simulink subsystem "forces"  (R2020a)
settings: Solver=VariableStepAuto  StartTime=0.0  StopTime=10.0  RelTol=1e-3
settings Model: Creator=Philip  LastModifiedBy=Philip

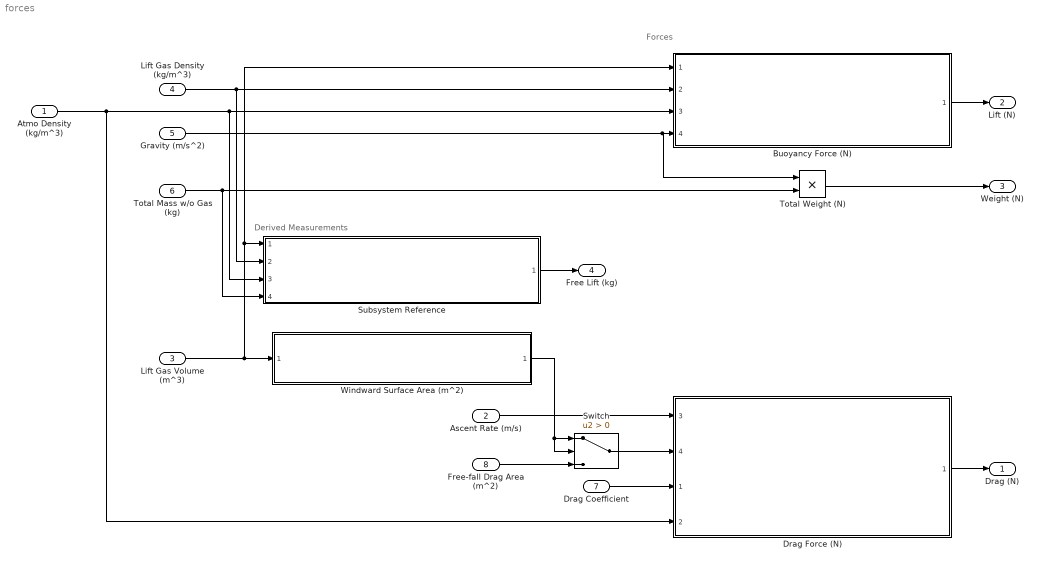
== system forces ==
  note: Forces
  note: Derived Measurements
  Atmo Density (kg/m^3) : Inport
  Ascent Rate (m/s) : Inport  Port=2
  Lift Gas Volume (m^3) : Inport  Port=3
  Lift Gas Density (kg/m^3) : Inport  Port=4
  Gravity (m/s^2) : Inport  Port=5
  Total Mass w/o Gas (kg) : Inport  Port=6
  Drag Coefficient : Inport  Port=7
  Free-fall Drag Area (m^2) : Inport  Port=8
  Buoyancy Force (N) : Subsystem  ReferencedSubsystem=buoyancy_force
  Drag Force (N) : Subsystem  ReferencedSubsystem=balloon_drag
      settings: PortSchema="{\"entries\":[{\"content\":{\"sides\":[{\"content\":{\"connectorIds\":[\"In3\",\"In4\",\"In1\",\"In2\"]},\"type\":\"ConnectorPlacement.EquallySpacedRectSide\",\"uuid\":\"149b4cde-76c5-4ca0-ad35-e24c4ea63904\"},{\"content\":{\"connectorIds\":[\"Out1\"],\"side\":\"RIGHT\"},\"type\":\"ConnectorPlacement.EquallySpacedRectSide\",\"uuid\":\"b3094bd8-666c-4796-b5f6-a24ca14a0216\"},{\"content\":{\"connectorIds\":[],\"side\":\"TOP\"},\"type\":\"ConnectorPlacement.EquallySpacedRectSide\",\"uuid\":\"8ef90c1d-a1d6-4cd7-a7b0-0fd7a3183b9f\"}]},\"type\":\"ConnectorPlacement.EquallySpacedConnector\",\"uuid\":\"ec47b48e-f4a0-4f5b-bade-ac3165f904c5\"}],\"packageUris\":[\"http://schema.mathworks.com/mf0/Connector/19700101\"],\"version\":\"1.0\"}"
  Subsystem Reference : Subsystem  ReferencedSubsystem=free_lift
  Switch : Switch  Criteria=u2 > Threshold
  Total Weight (N) : Product
  Windward Surface Area (m^2) : Subsystem  ReferencedSubsystem=balloon_drag_area
  Drag (N) : Outport
  Lift (N) : Outport  Port=2
  Weight (N) : Outport  Port=3
  Free Lift (kg) : Outport  Port=4
  wires:
  Subsystem Reference/1 -> Free Lift (kg)/1
  Lift Gas Density (kg/m^3)/1 -> Buoyancy Force (N)/2, Subsystem Reference/2
  Ascent Rate (m/s)/1 -> Drag Force (N)/3
  Drag Force (N)/1 -> Drag (N)/1
  Buoyancy Force (N)/1 -> Lift (N)/1
  Total Mass w/o Gas (kg)/1 -> Total Weight (N)/2, Subsystem Reference/4
  Total Weight (N)/1 -> Weight (N)/1
  Lift Gas Volume (m^3)/1 -> Windward Surface Area (m^2)/1, Subsystem Reference/1, Buoyancy Force (N)/1
  Atmo Density (kg/m^3)/1 -> Drag Force (N)/2, Buoyancy Force (N)/3, Subsystem Reference/3
  Gravity (m/s^2)/1 -> Buoyancy Force (N)/4, Total Weight (N)/1
  Windward Surface Area (m^2)/1 -> Switch/1, Switch/2
  Switch/1 -> Drag Force (N)/4
  Free-fall Drag Area (m^2)/1 -> Switch/3
  Drag Coefficient/1 -> Drag Force (N)/1
